simulink model "autopilot_total"  (R2021b)
settings: Solver=ode4  StartTime=0.0  StopTime=T  FixedStep=P.Ts  RelTol=1e-6  AbsTol=1e-3  EnableMultiTasking=on
values from neighbouring files (symbols this model uses):
  D = diag([0 k1*k3 k4/d])    [airspeedController.m]    (also in forces_moments.m; forces_moments_testing.m; precisionLanding.m)
  gama = 1    [airspeedController.m]    (also in forces_moments.m; forces_moments_testing.m; precisionLanding.m)
  k_VI = 0.8    [airspeedController.m]    (also in forces_moments.m; forces_moments_testing.m; main_precision_landing.m; precisionLanding.m)
  k_VP = 0.5    [airspeedController.m]    (also in forces_moments.m; forces_moments_testing.m; main_precision_landing.m; precisionLanding.m)
  mass = 25    [airspeedController.m]    (also in precisionLanding.m = P.mass)
undefined symbols (not defined in the file or in its folder): autopilot, forces_moments, gravity, P, true_states
libraries: simulink x3
settings Model: Creator=beard  LastModifiedBy=joaomoura
settings SolverCC: AutoScaleAbsTol=off  AlgebraicLoopSolver=TrustRegion
settings DataIOCC: LimitDataPoints=on  SaveFormat=Array  ReturnWorkspaceOutputs=off
settings OptimizationCC: ExpressionDepthLimit=2147483647  InitFltsAndDblsToZero=on  LifeSpan=inf
settings DebuggingCC: UnderspecifiedInitializationDetection=Classic  MergeDetectMultiDrivingBlocksExec=none  SolverPrmCheckMsg=warning  FcnCallInpInsideContextMsg=warning  StateNameClashWarn=warning  PregeneratedLibrarySubsystemCodeDiagnostic=none  SFUnexpectedBacktrackingDiag=warning  SFNoUnconditionalDefaultTransitionDiag=warning  SFExecutionAtInitializationDiag=none  SFMachineParentedDataDiag=warning  ArithmeticOperatorsInVariantConditions=warning
settings HardwareCC: ProdBitPerPointer=32  ProdBitPerSizeT=32  ProdBitPerPtrDiffT=32  ProdLargestAtomicFloat=None  ProdIntDivRoundTo=Undefined  ProdEndianess=Unspecified  ProdWordSize=32  ProdHWDeviceType=32-bit Generic
settings ModelReferenceCC: PropagateSignalLabelsOutOfModel=off
settings SFSimCC: SimUseLocalCustomCode=off  CustomCodeUndefinedFunction=UseInterfaceOnly
settings RTWCC: RTWUseLocalCustomCode=off
settings CodeAppCC: StateflowObjectComments=on
settings GRTTargetCC: TargetLangStandard=C89/C90 (ANSI)  CombineOutputUpdateFcns=off  GRTInterface=on
settings ConfigComp: CovMetricSettings=dw  CovSaveCumulativeToWorkspaceVar=on  CovSaveSingleToWorkspaceVar=on  CovExternalEMLEnable=off  CovSFcnEnable=off

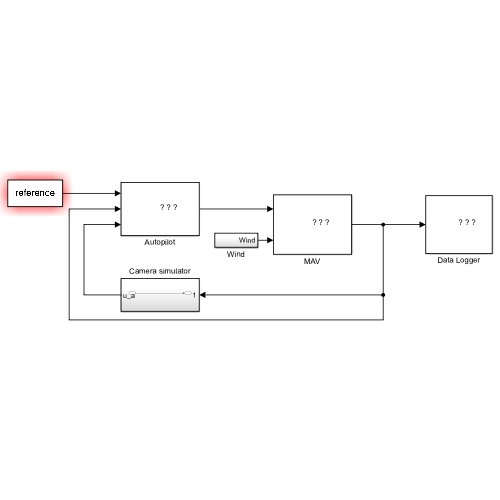
[thumbnail: Simulink's stored preview of the top-level diagram]
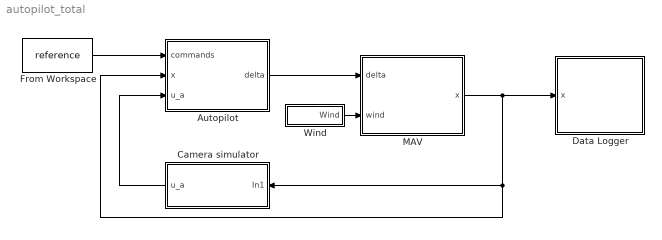
== system autopilot_total ==
  Autopilot : Subsystem
      mask Display: image(imread('simulink_imgs/kestrel.jpg'))
  Camera simulator : Subsystem
  Data Logger : Subsystem
      mask Display: image(imread('simulink_imgs/data_logger.png'))
  From Workspace : FromWorkspace  VariableName=reference
  MAV : Subsystem
      mask Display: image(imread('simulink_imgs/batcam.png'))
  Wind : Subsystem
  wires:
  Wind/1(Wind) -> MAV/2(wind)
  MAV/1(x) -> Data Logger/1(x), Camera simulator/1(In1), Autopilot/2(x)
  Autopilot/1(delta) -> MAV/1(delta)
  From Workspace/1 -> Autopilot/1(commands)
  Camera simulator/1(u_a) -> Autopilot/3(u_a)

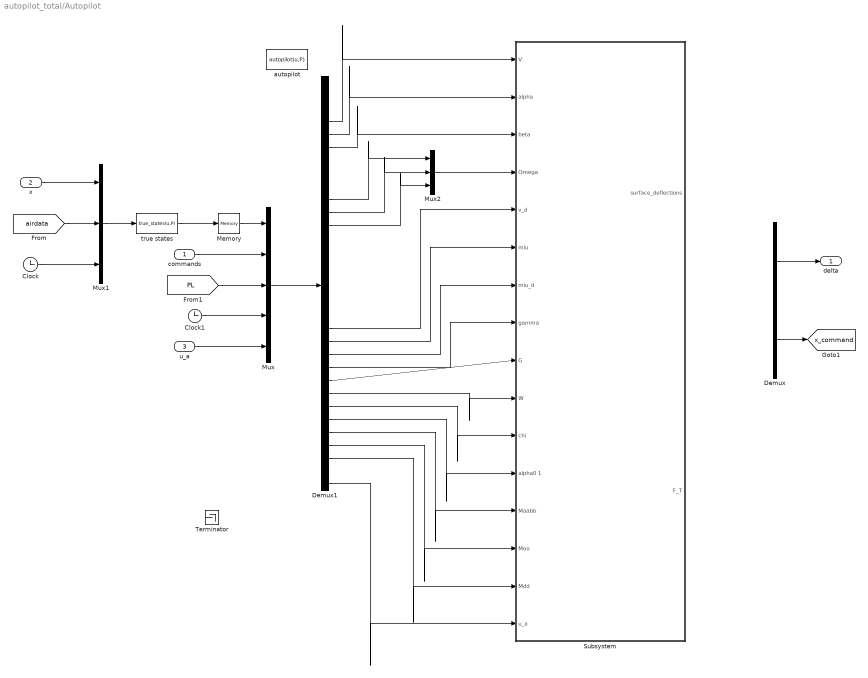
== system autopilot_total/Autopilot ==
  commands : Inport
  x : Inport  Port=2
  u_a : Inport  Port=3
  Clock : Clock
  Clock1 : Clock
  Demux : Demux  Outputs=[4;2]
  Demux1 : Demux  Outputs=19+1+10+1+1
  Memory : Memory
  Mux : Mux  Inputs=5
  Mux1 : Mux  Inputs=3
  Mux2 : Mux  Inputs=3
  Subsystem : Subsystem
  Terminator : Terminator
  autopilot : MATLABFcn  MATLABFcn=autopilot(u,P)  OutputDimensions=4+2  SampleTime=P.Ts
  true states : MATLABFcn  MATLABFcn=true_states(u,P)  OutputDimensions=19  SampleTime=P.Ts
  delta : Outport  VectorParamsAs1DForOutWhenUnconnected=off
  tag scope: x_command=global
  wires:
  Clock/1 -> Mux1/3
  Demux/1 -> delta/1
  Demux/2 -> [x_command]
  commands/1 -> Mux/2
  Mux1/1 -> true states/1
  x/1 -> Mux1/1
  true states/1 -> Memory/1
  [airdata] -> Mux1/2
  Memory/1 -> Mux/1
  Clock1/1 -> Mux/4
  [PL] -> Mux/3
  Mux/1 -> Demux1/1
  Demux1/4 -> Subsystem/1(V)
  Demux1/5 -> Subsystem/2(alpha)
  Demux1/6 -> Subsystem/3(beta)
  Demux1/20 -> Subsystem/5(v_d)
  Demux1/10 -> Mux2/1
  Demux1/11 -> Mux2/2
  Demux1/12 -> Mux2/3
  Mux2/1 -> Subsystem/4("Omega ")
  Demux1/21 -> Subsystem/6(miu)
  Demux1/22 -> Subsystem/7(miu_d)
  Demux1/23 -> Subsystem/8(gamma)
  Demux1/24 -> Subsystem/9(G)
  Demux1/25 -> Subsystem/10(W)
  u_a/1 -> Mux/5
  Demux1/26 -> Subsystem/11(chi)
  Demux1/27 -> Subsystem/12(alpha0 1)
  Demux1/28 -> Subsystem/13(Maabb)
  Demux1/29 -> Subsystem/14(Moo)
  Demux1/30 -> Subsystem/15(Mdd)
  Demux1/32 -> Subsystem/16(u_a)

== system autopilot_total/Camera simulator ==
  In1 : Inport
  u_a : Outport
  wires:
  In1/1 -> u_a/1

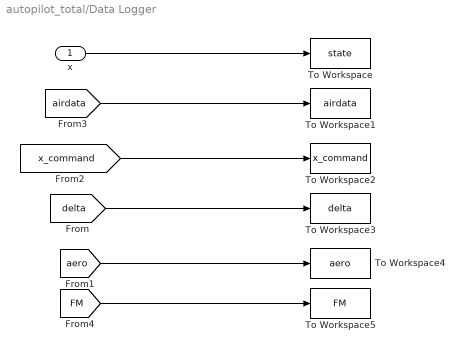
== system autopilot_total/Data Logger ==
  x : Inport
  To Workspace : ToWorkspace  VariableName=state  SaveFormat=Structure With Time  SampleTime=-1
  To Workspace1 : ToWorkspace  VariableName=airdata  SaveFormat=Structure With Time  SampleTime=-1
  To Workspace2 : ToWorkspace  VariableName=x_command  SaveFormat=Structure With Time  SampleTime=-1
  To Workspace3 : ToWorkspace  VariableName=delta  SaveFormat=Structure With Time  SampleTime=-1
  To Workspace4 : ToWorkspace  VariableName=aero  SaveFormat=Structure With Time  SampleTime=-1
  To Workspace5 : ToWorkspace  VariableName=FM  SaveFormat=Structure With Time  SampleTime=-1
  wires:
  x/1 -> To Workspace/1
  [x_command] -> To Workspace2/1
  [delta] -> To Workspace3/1
  [airdata] -> To Workspace1/1
  [aero] -> To Workspace4/1
  [FM] -> To Workspace5/1

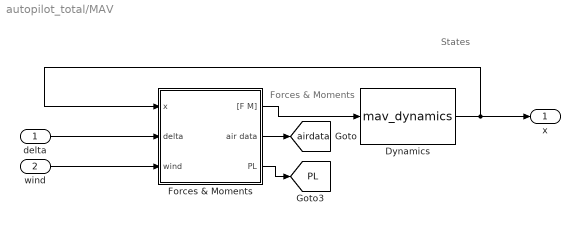
== system autopilot_total/MAV ==
  note: Forces & Moments
  note: States
  delta : Inport
  wind : Inport  Port=2
  Dynamics : S-Function  FunctionName=mav_dynamics  Parameters=P  SFunctionDeploymentMode=off  EnableBusSupport=off
  Forces & Moments : Subsystem
  x : Outport  VectorParamsAs1DForOutWhenUnconnected=off
  tag scope: PL=global, airdata=global
  wires:
  Dynamics/1 -> Forces & Moments/1(x), x/1
  Forces & Moments/1("[F M]") -> Dynamics/1
  Forces & Moments/2(air data) -> [airdata]
  delta/1 -> Forces & Moments/2(delta)
  wind/1 -> Forces & Moments/3(wind)
  Forces & Moments/3(PL) -> [PL]

== system autopilot_total/Wind ==
  Constant2 : Constant  Value=[P.wind_n; P.wind_e; P.wind_d]
  Mux1 : Mux  Inputs=2
  Wind Gusts : Subsystem
  Wind : Outport  VectorParamsAs1DForOutWhenUnconnected=off
  wires:
  Constant2/1 -> Mux1/1
  Mux1/1 -> Wind/1
  Wind Gusts/1(gusts) -> Mux1/2

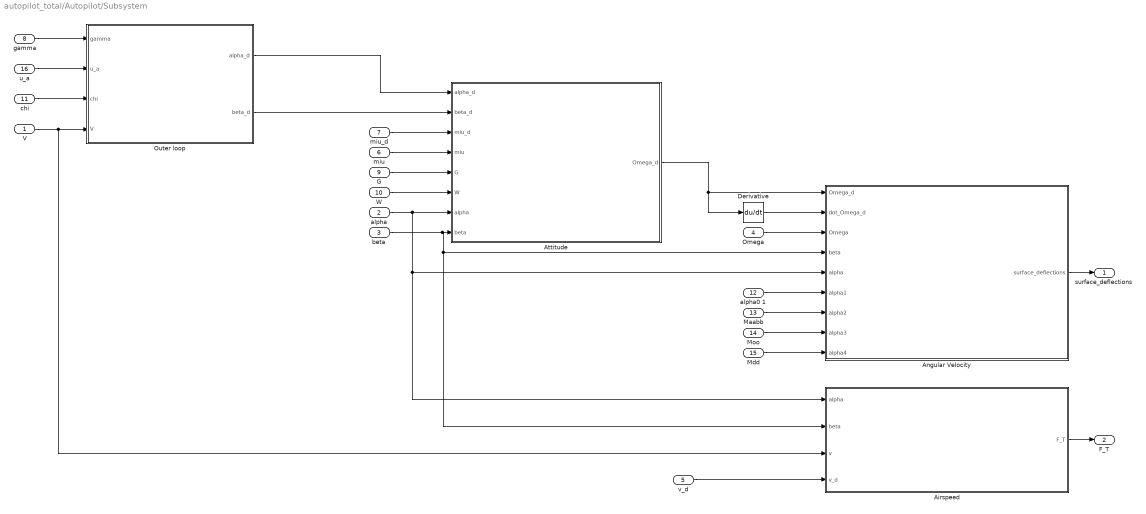
== system autopilot_total/Autopilot/Subsystem ==
  V : Inport
  alpha : Inport  Port=2
  beta : Inport  Port=3
  "Omega " : Inport  Port=4
  v_d : Inport  Port=5
  miu : Inport  Port=6
  miu_d : Inport  Port=7
  gamma : Inport  Port=8
  G : Inport  Port=9
  W : Inport  Port=10
  chi : Inport  Port=11
  alpha0 1 : Inport  Port=12
  Maabb : Inport  Port=13
  Moo : Inport  Port=14
  Mdd : Inport  Port=15
  u_a : Inport  Port=16
  Airspeed : Subsystem
  Angular Velocity : Subsystem
  Attitude : Subsystem
  Derivative : Derivative
  Outer loop : Subsystem
  surface_deflections : Outport  VectorParamsAs1DForOutWhenUnconnected=off
  "F_T " : Outport  Port=2  VectorParamsAs1DForOutWhenUnconnected=off
  wires:
  Attitude/1(Omega_d) -> Derivative/1, Angular Velocity/1(Omega_d)
  Outer loop/2(beta_d) -> Attitude/2(beta_d)
  v_d/1 -> Airspeed/4(v_d)
  gamma/1 -> Outer loop/1(gamma)
  Airspeed/1("F_T ") -> "F_T "/1
  "Omega "/1 -> Angular Velocity/3(Omega)
  miu/1 -> Attitude/4(miu)
  beta/1 -> Airspeed/2(beta), Angular Velocity/4(beta), Attitude/8(beta)
  miu_d/1 -> Attitude/3(miu_d)
  Outer loop/1(alpha_d) -> Attitude/1(alpha_d)
  V/1 -> Outer loop/4(V), Airspeed/3("v ")
  Angular Velocity/1(surface_deflections) -> surface_deflections/1
  alpha/1 -> Attitude/7(alpha), Airspeed/1(alpha), Angular Velocity/5(alpha)
  u_a/1 -> Outer loop/2(u_a)
  chi/1 -> Outer loop/3(chi)
  Derivative/1 -> Angular Velocity/2(dot_Omega_d)
  G/1 -> Attitude/5(G)
  W/1 -> Attitude/6(W)
  alpha0 1/1 -> Angular Velocity/6(alpha1)
  Maabb/1 -> Angular Velocity/7(alpha2)
  Moo/1 -> Angular Velocity/8(alpha3)
  Mdd/1 -> Angular Velocity/9(alpha4)

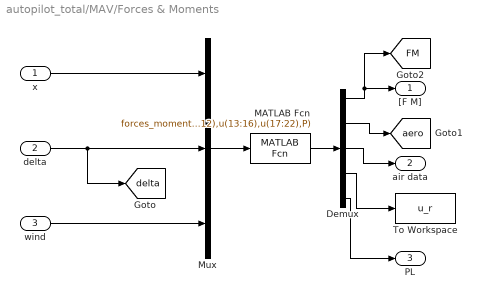
== system autopilot_total/MAV/Forces & Moments ==
  x : Inport
  delta : Inport  Port=2
  wind : Inport  Port=3
  Demux : Demux  Outputs=[6;6;6;1;8]
  MATLAB Fcn : MATLABFcn  MATLABFcn=forces_moments(u(1:12),u(13:16),u(17:22),P)  OutputDimensions=19
  Mux : Mux  Inputs=3
  To Workspace : ToWorkspace  VariableName=u_r  SampleTime=-1
  "[F M]" : Outport  VectorParamsAs1DForOutWhenUnconnected=off
  air data : Outport  Port=2  VectorParamsAs1DForOutWhenUnconnected=off
  PL : Outport  Port=3  VectorParamsAs1DForOutWhenUnconnected=off
  tag scope: FM=global, aero=global, delta=global
  wires:
  Mux/1 -> MATLAB Fcn/1
  Demux/1 -> [FM], "[F M]"/1
  MATLAB Fcn/1 -> Demux/1
  wind/1 -> Mux/3
  delta/1 -> Mux/2, [delta]
  x/1 -> Mux/1
  Demux/3 -> air data/1
  Demux/2 -> [aero]
  Demux/4 -> To Workspace/1
  Demux/5 -> PL/1

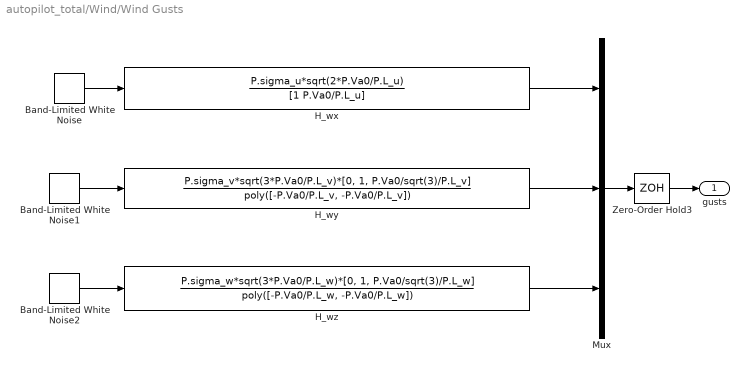
== system autopilot_total/Wind/Wind Gusts ==
  Band-Limited White Noise : simulink/Sources/Band-Limited White Noise  Cov=[1]  Ts=P.Ts  seed=[23341]
  Band-Limited White Noise1 : simulink/Sources/Band-Limited White Noise  Cov=[1]  Ts=P.Ts  seed=[23341]
  Band-Limited White Noise2 : simulink/Sources/Band-Limited White Noise  Cov=[1]  Ts=P.Ts  seed=[23341]
  H_wx : TransferFcn  Numerator=P.sigma_u*sqrt(2*P.Va0/P.L_u)  Denominator=[1 P.Va0/P.L_u]
  H_wy : TransferFcn  Numerator=P.sigma_v*sqrt(3*P.Va0/P.L_v)*[0, 1, P.Va0/sqrt(3)/P.L_v]  Denominator=poly([-P.Va0/P.L_v, -P.Va0/P.L_v])
  H_wz : TransferFcn  Numerator=P.sigma_w*sqrt(3*P.Va0/P.L_w)*[0, 1, P.Va0/sqrt(3)/P.L_w]  Denominator=poly([-P.Va0/P.L_w, -P.Va0/P.L_w])
  Mux : Mux  Inputs=3
  Zero-Order Hold3 : ZeroOrderHold  SampleTime=P.Ts
  gusts : Outport  VectorParamsAs1DForOutWhenUnconnected=off
  wires:
  H_wx/1 -> Mux/1
  Band-Limited White Noise/1 -> H_wx/1
  H_wy/1 -> Mux/2
  Band-Limited White Noise1/1 -> H_wy/1
  H_wz/1 -> Mux/3
  Band-Limited White Noise2/1 -> H_wz/1
  Mux/1 -> Zero-Order Hold3/1
  Zero-Order Hold3/1 -> gusts/1

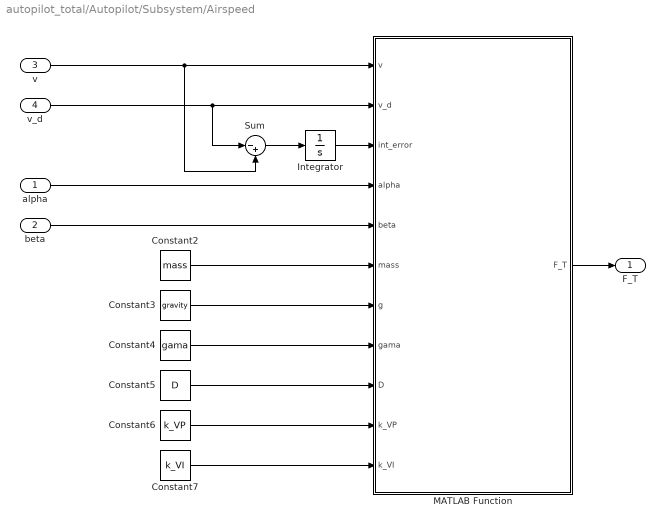
== system autopilot_total/Autopilot/Subsystem/Airspeed ==
  alpha : Inport
  beta : Inport  Port=2
  "v " : Inport  Port=3
  v_d : Inport  Port=4
  Constant2 : Constant  Value=mass
  Constant3 : Constant  Value=gravity
  Constant4 : Constant  Value=gama
  Constant5 : Constant  Value=D
  Constant6 : Constant  Value=k_VP
  Constant7 : Constant  Value=k_VI
  Integrator : Integrator
  MATLAB Function : MATLAB Function  TreatAsAtomicUnit=on
  Sum : Sum  Inputs=|-+
  "F_T " : Outport  VectorParamsAs1DForOutWhenUnconnected=off
  wires:
  Constant3/1 -> MATLAB Function/7(g)
  v_d/1 -> Sum/1, MATLAB Function/2(v_d)
  Constant4/1 -> MATLAB Function/8(gama)
  Constant7/1 -> MATLAB Function/11(k_VI)
  beta/1 -> MATLAB Function/5(beta)
  Constant5/1 -> MATLAB Function/9(D)
  Constant6/1 -> MATLAB Function/10(k_VP)
  MATLAB Function/1(F_T) -> "F_T "/1
  "v "/1 -> Sum/2, MATLAB Function/1(v)
  Integrator/1 -> MATLAB Function/3(int_error)
  alpha/1 -> MATLAB Function/4(alpha)
  Sum/1 -> Integrator/1
  Constant2/1 -> MATLAB Function/6(mass)

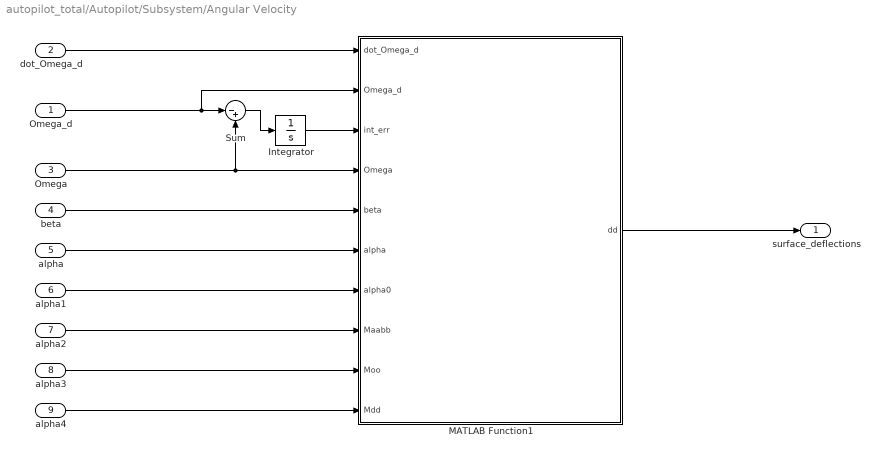
== system autopilot_total/Autopilot/Subsystem/Angular Velocity ==
  Omega_d : Inport
  dot_Omega_d : Inport  Port=2
  Omega : Inport  Port=3
  beta : Inport  Port=4
  alpha : Inport  Port=5
  alpha1 : Inport  Port=6
  alpha2 : Inport  Port=7
  alpha3 : Inport  Port=8
  alpha4 : Inport  Port=9
  Integrator : Integrator
  MATLAB Function1 : MATLAB Function  TreatAsAtomicUnit=on
  Sum : Sum  Inputs=|-+
  surface_deflections : Outport  VectorParamsAs1DForOutWhenUnconnected=off
  wires:
  alpha2/1 -> MATLAB Function1/8(Maabb)
  Omega_d/1 -> MATLAB Function1/2(Omega_d), Sum/1
  Sum/1 -> Integrator/1
  alpha4/1 -> MATLAB Function1/10(Mdd)
  dot_Omega_d/1 -> MATLAB Function1/1(dot_Omega_d)
  beta/1 -> MATLAB Function1/5(beta)
  Omega/1 -> Sum/2, MATLAB Function1/4(Omega)
  alpha3/1 -> MATLAB Function1/9(Moo)
  alpha1/1 -> MATLAB Function1/7(alpha0)
  Integrator/1 -> MATLAB Function1/3(int_err)
  MATLAB Function1/1(dd) -> surface_deflections/1
  alpha/1 -> MATLAB Function1/6(alpha)

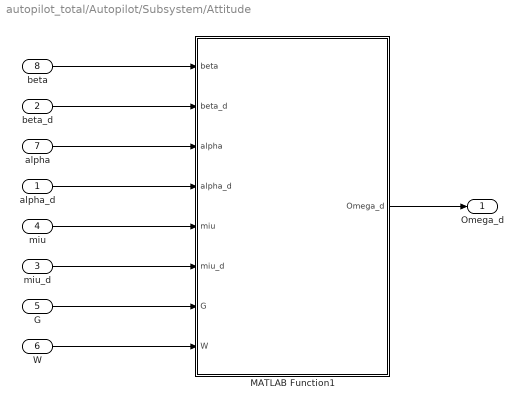
== system autopilot_total/Autopilot/Subsystem/Attitude ==
  alpha_d : Inport
  beta_d : Inport  Port=2
  miu_d : Inport  Port=3
  miu : Inport  Port=4
  G : Inport  Port=5
  W : Inport  Port=6
  alpha : Inport  Port=7
  beta : Inport  Port=8
  MATLAB Function1 : MATLAB Function  TreatAsAtomicUnit=on
  Omega_d : Outport  VectorParamsAs1DForOutWhenUnconnected=off
  wires:
  MATLAB Function1/1(Omega_d) -> Omega_d/1
  alpha_d/1 -> MATLAB Function1/4(alpha_d)
  beta_d/1 -> MATLAB Function1/2(beta_d)
  miu_d/1 -> MATLAB Function1/6(miu_d)
  miu/1 -> MATLAB Function1/5(miu)
  beta/1 -> MATLAB Function1/1(beta)
  alpha/1 -> MATLAB Function1/3(alpha)
  G/1 -> MATLAB Function1/7(G)
  W/1 -> MATLAB Function1/8(W)

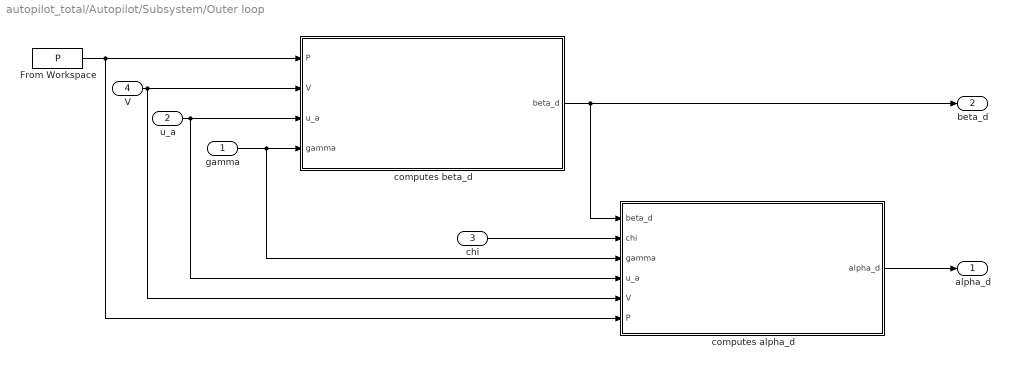
== system autopilot_total/Autopilot/Subsystem/Outer loop ==
  gamma : Inport
  u_a : Inport  Port=2
  chi : Inport  Port=3
  V : Inport  Port=4
  From Workspace : FromWorkspace  VariableName=P
  computes alpha_d : Subsystem
  computes beta_d : Subsystem
  alpha_d : Outport
  beta_d : Outport  Port=2
  wires:
  computes beta_d/1(beta_d) -> computes alpha_d/1(beta_d), beta_d/1
  computes alpha_d/1(alpha_d) -> alpha_d/1
  gamma/1 -> computes alpha_d/3(gamma), computes beta_d/4(gamma)
  u_a/1 -> computes beta_d/3(u_a), computes alpha_d/4(u_a)
  chi/1 -> computes alpha_d/2(chi)
  From Workspace/1 -> computes alpha_d/6(P), computes beta_d/1(P)
  V/1 -> computes beta_d/2(V), computes alpha_d/5(V)

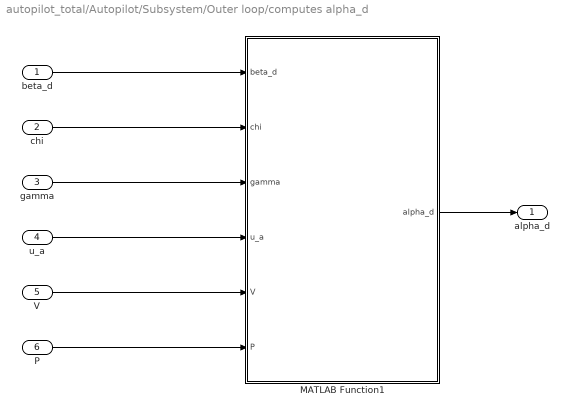
== system autopilot_total/Autopilot/Subsystem/Outer loop/computes alpha_d ==
  beta_d : Inport
  chi : Inport  Port=2
  gamma : Inport  Port=3
  u_a : Inport  Port=4
  V : Inport  Port=5
  P : Inport  Port=6
  MATLAB Function1 : MATLAB Function  TreatAsAtomicUnit=on
  alpha_d : Outport  VectorParamsAs1DForOutWhenUnconnected=off
  wires:
  MATLAB Function1/1(alpha_d) -> alpha_d/1
  beta_d/1 -> MATLAB Function1/1(beta_d)
  P/1 -> MATLAB Function1/6(P)
  u_a/1 -> MATLAB Function1/4(u_a)
  chi/1 -> MATLAB Function1/2(chi)
  gamma/1 -> MATLAB Function1/3(gamma)
  V/1 -> MATLAB Function1/5(V)

== system autopilot_total/Autopilot/Subsystem/Outer loop/computes beta_d ==
  P : Inport
  V : Inport  Port=2
  u_a : Inport  Port=3
  gamma : Inport  Port=4
  MATLAB Function1 : MATLAB Function  TreatAsAtomicUnit=on
  beta_d : Outport  VectorParamsAs1DForOutWhenUnconnected=off
  wires:
  MATLAB Function1/1(beta_d) -> beta_d/1
  P/1 -> MATLAB Function1/1(P)
  u_a/1 -> MATLAB Function1/3(u_a)
  gamma/1 -> MATLAB Function1/4(gamma)
  V/1 -> MATLAB Function1/2(V)

== matlab function autopilot_total/Autopilot/Subsystem/Airspeed/MATLAB Function ==
  data: v input; v_d input; F_T output; int_error input; alpha input; beta input; mass input; g input; gama input; D input; k_VP input; k_VI input
function F_T = airspeedController(v,v_d,int_error,alpha,beta,mass,g,gama,D,k_VP,k_VI)
% Equation 47 [1]

F_T = [(D + mass*g*sin(gama)/(cos(beta)*cos(alpha))] + ...
      [(k_VP*(v-v_d) + k_VI*int_error)/(cos(beta)*cos(alpha))];

end

% [1] Serra, Pedro & Cunha, Rita & Hamel, T. & Silvestre, Carlos & Le Bras, Florent. (2015). Nonlinear Image-Based Visual Servo Controller for the Flare Maneuver of Fixed-Wing Aircraft Using Optical Flow. IEEE Transactions on Control Systems Technology. 23. 570–583. 10.1109/TCST.2014.2330996.

== matlab function autopilot_total/Autopilot/Subsystem/Angular Velocity/MATLAB Function1 ==
  data: dot_Omega_d input; Omega_d input; int_err input; Omega input; beta input; alpha input; alpha0 input; Maabb input; dd output; Moo input; Mdd input
function dd = controller(dot_Omega_d,Omega_d,int_err,Omega,beta,alpha,alpha0,Maabb,Moo,Mdd)
% Equation 48 [1]

    % gains
    kp = 1;
    ki = 1;
    
    % auxiliary calculations
    Soo = skew(Omega);
    
    % control law
    dd = Mdd\(Soo*Omega-...
        Maabb*[beta;alpha-alpha0]-...
        Moo*Omega-...
        kp*(Omega-Omega_d)-...
        ki*int_err+dot_Omega_d);
end

function S = skew(vector)
    S = [0,-vector(3),vector(2);
        vector(3),0,-vector(1);
        -vector(2),vector(1),0];
end

% [1] Serra, Pedro & Cunha, Rita & Hamel, T. & Silvestre, Carlos & Le Bras, Florent. (2015). Nonlinear Image-Based Visual Servo Controller for the Flare Maneuver of Fixed-Wing Aircraft Using Optical Flow. IEEE Transactions on Control Systems Technology. 23. 570–583. 10.1109/TCST.2014.2330996.

== matlab function autopilot_total/Autopilot/Subsystem/Attitude/MATLAB Function1 ==
  data: beta input; beta_d input; alpha input; alpha_d input; miu input; miu_d input; G input; Omega_d output; W input
function Omega_d = controller(beta,beta_d,alpha,alpha_d,miu,miu_d,G,W)

    % gains
    Kp = 1;
    
    % control law
    Omega_d = G\(-W-Kp*[beta-beta_d;alpha-alpha_d;miu-miu_d]);
end

== matlab function autopilot_total/Autopilot/Subsystem/Outer loop/computes alpha_d/MATLAB Function1 ==
  data: beta_d input; chi input; gamma input; u_a input; V input; P input; alpha_d output
function alpha_d = controller(beta_d,chi,gamma,u_a,V,P)
    
    
    % params
    q_bar = 0.5*P.rho*V^2;

    ad1 = q_bar * P.S_wing * P.C_D_alpha;
    ad2 = q_bar * P.S_wing * (CL_alpha + P.C_D_0 - P.C_Y_beta * beta_d * tan(beta_d))...
        + m*g * sin(gamma) * 1/cos(beta_d);

    ad3 = -P.mass*P.gravity*cos(gamma) + q_bar*P.S_wing*P.C_L_0 - [0;1;0] * u_a/cos(chi);

    % control law

    alpha_d = (-ad2 + sqrt(ad2^2-4*ad1*ad3))/(2*ad1);

end


% duvida: na equação no paper (ultima pagina) tem la: Cl0_linha e Cd0_linha
% e nao Cl0 e Cd0, no entanto não se fala mais desses parâmetros (com
% linha) no paper e nós também não temos isso e eu nao sei o que é

== matlab function autopilot_total/Autopilot/Subsystem/Outer loop/computes beta_d/MATLAB Function1 ==
  data: P input; V input; u_a input; gamma input; beta_d output
function beta_d = controller(P,V,u_a,gamma)
    % params
    q_bar = 0.5*P.rho*V^2;
    
    % control law

    beta_d = ([0;0;1]*u_a*cos(gamma)) / (q_bar*S*P.C_Y_beta - P.mass*P.gravity*sin(gamma));

end
